simulink model "controle_2018a"  (R2018a)
settings: Solver=FixedStepAuto  StartTime=0.0  StopTime=2000  FixedStep=0.01  RelTol=1e-3
libraries: neural x39, simulink x6
(part 2 of 2)

== system controle_2018a/Feed-Forward Neural Network/Layer 4/Delays 1 ==
  "p{4}" : Inport  PortDimensions=20
      mask Display: e = 0.06;c1 = [120 230 180]/255;c2 = ([120 230 180]+0)/(256+128);c3 = ([120 230 180]+128)/(256+128);patch([0 1 1 0],[0 0 1 1],c1);patch([0 1 1 1-e 1-e 0+e],[0 0 1 1-e 0+e 0+e],c2);patch([0 0 1 1-e 0+e 0+e],[0 1 1 1-e 1-e 0+e],c3);plot([0 1 1 0 0],[0 0 1 1 0]);
  mux : Mux  Inputs=1
      mask Display: e = 0.06;c1 = [120 150 230]/255;c2 = ([120 150 230]+0)/383;c3 = ([120 150 230]+128)/383;patch([0 1 1 0],[0 0 1 1],c1);patch([0 1 1 1-e 1-e 0+e],[0 0 1 1-e 0+e 0+e],c2);patch([0 0 1 1-e 0+e 0+e],[0 1 1 1-e 1-e 0+e],c3);plot([0 1 1 0 0],[0 0 1 1 0]);disp('Mux')
  "pd{4,3}" : Outport
      mask Display: e = 0.06;c1 = [120 230 180]/255;c2 = ([120 230 180]+0)/(256+128);c3 = ([120 230 180]+128)/(256+128);patch([0 1 1 0],[0 0 1 1],c1);patch([0 1 1 1-e 1-e 0+e],[0 0 1 1-e 0+e 0+e],c2);patch([0 0 1 1-e 0+e 0+e],[0 1 1 1-e 1-e 0+e],c3);plot([0 1 1 0 0],[0 0 1 1 0]);
  wires:
  mux/1 -> "pd{4,3}"/1
  "p{4}"/1 -> mux/1

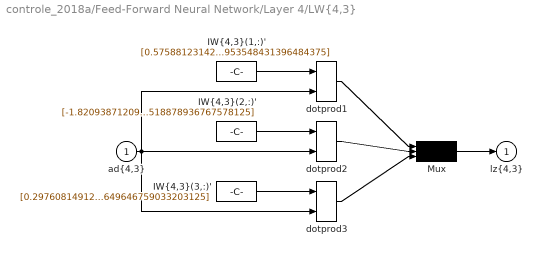
== system controle_2018a/Feed-Forward Neural Network/Layer 4/LW{4,3} ==
  "ad{4,3}" : Inport  PortDimensions=20
      mask Display: e = 0.06;c1 = [120 230 180]/255;c2 = ([120 230 180]+0)/(256+128);c3 = ([120 230 180]+128)/(256+128);patch([0 1 1 0],[0 0 1 1],c1);patch([0 1 1 1-e 1-e 0+e],[0 0 1 1-e 0+e 0+e],c2);patch([0 0 1 1-e 0+e 0+e],[0 1 1 1-e 1-e 0+e],c3);plot([0 1 1 0 0],[0 0 1 1 0]);
  "IW{4,3}(1,:)'" : Constant  Value=[0.5758812314286243516647800788632594048976898193359375;2.763204978975422942966133632580749690532684326171875;-1.2802722053804782564867537075770087540149688720703125;1.0039832432065936007603568214108236134052276611328125;0.8258444763193881765772630387800745666027069091796875;-1.09338814333258138589144436991773545742034912109375;-0.2477185626340651924959246343860286287963390350341796875;-0.395941672531393951128819708173978142440319061279296875;-0.4377604585731760256095412842114455997943878173828125;-0.95218991269365493845810988204902969300746917724609375;0.6590241743146219022264631348662078380584716796875;-0.00786928649653931104601678470089609618298709392547607421875;-0.220411098181123310535411974342423491179943084716796875;0.88687130330759267327067618680302985012531280517578125;-0.3596937800311688082643968300544656813144683837890625;1.2121688518179885019065977758145891129970550537109375;-0.438603936560962914814609803215716965496540069580078125;-0.417442181161946923584338264845428057014942169189453125;0.0477252038977766523952794841534341685473918914794921875;-0.844130604200289180738536742865107953548431396484375]
      mask Display: e = 0.06;c1 = [120 150 230]/255;c2 = ([120 150 230]+0)/383;c3 = ([120 150 230]+128)/383;patch([0 1 1 0],[0 0 1 1],c1);patch([0 1 1 1-e 1-e 0+e],[0 0 1 1-e 0+e 0+e],c2);patch([0 0 1 1-e 0+e 0+e],[0 1 1 1-e 1-e 0+e],c3);plot([0 1 1 0 0],[0 0 1 1 0]);disp('weights');
  "IW{4,3}(2,:)'" : Constant  Value=[-1.82093871209123125964879363891668617725372314453125;3.331995899235053126830052860896103084087371826171875;0.8720127611111958554346301752957515418529510498046875;-0.1215641173061823565593186913247336633503437042236328125;0.97129900070614727525253329076804220676422119140625;-0.66265929292588021670695752618485130369663238525390625;-1.455057403808262872502155005349777638912200927734375;-0.26820688469812381526935496367514133453369140625;0.5972049607486102917874859485891647636890411376953125;-1.7138306843531510015310459493775852024555206298828125;-1.351996426070770862537528955726884305477142333984375;0.2082923649721768744047523114204523153603076934814453125;-0.85504087835445841125903143620234914124011993408203125;0.7048199503255430098391798310331068933010101318359375;0.310425306529726052762185872779809869825839996337890625;-0.04836223927535530930921225944985053502023220062255859375;0.80016323569060343601222484721802175045013427734375;-1.0380612236424358041375626271474175155162811279296875;0.061202250631397780988862677986617200076580047607421875;0.13788600142726814556937142697279341518878936767578125]
      mask Display: e = 0.06;c1 = [120 150 230]/255;c2 = ([120 150 230]+0)/383;c3 = ([120 150 230]+128)/383;patch([0 1 1 0],[0 0 1 1],c1);patch([0 1 1 1-e 1-e 0+e],[0 0 1 1-e 0+e 0+e],c2);patch([0 0 1 1-e 0+e 0+e],[0 1 1 1-e 1-e 0+e],c3);plot([0 1 1 0 0],[0 0 1 1 0]);disp('weights');
  "IW{4,3}(3,:)'" : Constant  Value=[0.297608149129080568062732936596148647367954254150390625;0.413239085577538578508693944968399591743946075439453125;-0.792515163261203081646044665831141173839569091796875;-2.2444387000121803765750883030705153942108154296875;0.542372050978492392658836251939646899700164794921875;0.92716028959430218936432765985955484211444854736328125;1.0742093909963810194341249371063895523548126220703125;-0.46873953716529437318882855834090150892734527587890625;-0.323837139828971221078290909645147621631622314453125;0.79374999139544344384233909295289777219295501708984375;0.09925135785478327032915757399678113870322704315185546875;0.38166887655685044489217716545681469142436981201171875;1.78278709879469676735652683419175446033477783203125;0.01781218307202965533964089672736008651554584503173828125;1.034664848416760651872436937992461025714874267578125;-0.6548703206903943030425807592109777033329010009765625;0.194469801477239523368467644104384817183017730712890625;0.400177509632150651963655718645895831286907196044921875;1.3097456202543913406088904594071209430694580078125;-0.1597640871039971710576566010786336846649646759033203125]
      mask Display: e = 0.06;c1 = [120 150 230]/255;c2 = ([120 150 230]+0)/383;c3 = ([120 150 230]+128)/383;patch([0 1 1 0],[0 0 1 1],c1);patch([0 1 1 1-e 1-e 0+e],[0 0 1 1-e 0+e 0+e],c2);patch([0 0 1 1-e 0+e 0+e],[0 1 1 1-e 1-e 0+e],c3);plot([0 1 1 0 0],[0 0 1 1 0]);disp('weights');
  Mux : Mux  Inputs=3
      mask Display: e = 0.06;c1 = [120 150 230]/255;c2 = ([120 150 230]+0)/383;c3 = ([120 150 230]+128)/383;patch([0 1 1 0],[0 0 1 1],c1);patch([0 1 1 1-e 1-e 0+e],[0 0 1 1-e 0+e 0+e],c2);patch([0 0 1 1-e 0+e 0+e],[0 1 1 1-e 1-e 0+e],c3);plot([0 1 1 0 0],[0 0 1 1 0]);disp('Mux');
  dotprod1 : neural/Weight Functions/dotprod
  dotprod2 : neural/Weight Functions/dotprod
  dotprod3 : neural/Weight Functions/dotprod
  "lz{4,3}" : Outport
      mask Display: e = 0.06;c1 = [120 230 180]/255;c2 = ([120 230 180]+0)/(256+128);c3 = ([120 230 180]+128)/(256+128);patch([0 1 1 0],[0 0 1 1],c1);patch([0 1 1 1-e 1-e 0+e],[0 0 1 1-e 0+e 0+e],c2);patch([0 0 1 1-e 0+e 0+e],[0 1 1 1-e 1-e 0+e],c3);plot([0 1 1 0 0],[0 0 1 1 0]);
  wires:
  Mux/1 -> "lz{4,3}"/1
  dotprod3/1 -> Mux/3
  "IW{4,3}(3,:)'"/1 -> dotprod3/1
  dotprod2/1 -> Mux/2
  "IW{4,3}(2,:)'"/1 -> dotprod2/1
  dotprod1/1 -> Mux/1
  "ad{4,3}"/1 -> dotprod3/2, dotprod2/2, dotprod1/2
  "IW{4,3}(1,:)'"/1 -> dotprod1/1

== matlab function controle_2018a/camera ==
  data: x output; output input; y output; z output
function [x,y,z] = robo(output)

% Manda info pro arduino
% Adquire posicao com camera

x = output(1);
y = output(2);
z = output(3);
end
